simulink model "Model"  (R2020b)
settings: Solver=FixedStepAuto  StartTime=0.0  StopTime=40  FixedStep=0.01  RelTol=1e-3
undefined symbols (not defined in the file or in its folder): DiscIntNeverNeededParam, drv, g, gbox, lqr_integral, lqr_nominal, ms22g, nlmodel, Nu, Nx, sens, stvar_est, Ts, wheel, x01
settings Model: Creator=Utente  LastModifiedBy=pellizzar1

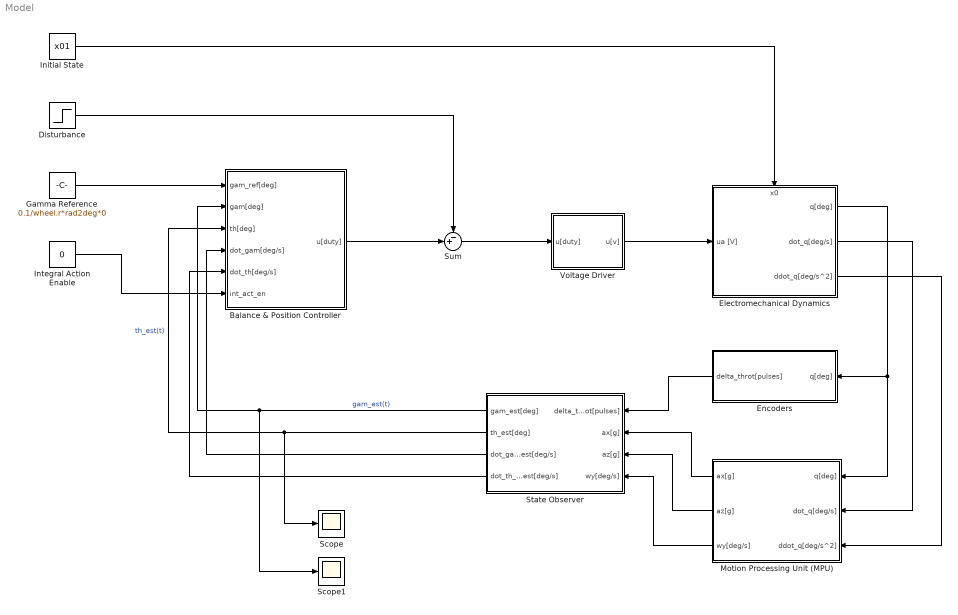
== system Model ==
  Balance & Position Controller : Subsystem
  Disturbance : Step  Time=10  After=5.0/drv.duty2V*0  SampleTime=0
  Electromechanical Dynamics : Subsystem
      settings: PortSchema="{\"entries\":[{\"content\":{\"sides\":[{\"content\":{\"connectorIds\":[\"In1\"]},\"type\":\"ConnectorPlacement.EquallySpacedRectSide\",\"uuid\":\"048a8cca-500e-4f29-b02e-3058ec048dc6\"},{\"content\":{\"connectorIds\":[\"Out1\",\"Out2\",\"Out3\"],\"side\":\"RIGHT\"},\"type\":\"ConnectorPlacement.EquallySpacedRectSide\",\"uuid\":\"804c427c-9fad-47de-8a12-f7821be643d3\"},{\"content\":{\"connectorIds\":[\"In2\"],\"side\":\"TOP\"},\"type\":\"ConnectorPlacement.EquallySpacedRectSide\",\"uuid\":\"0670649b-5041-4c19-9bef-d5e2c260ec4c\"},{\"content\":{\"connectorIds\":[],\"side\":\"HIDDEN\"},\"type\":\"ConnectorPlacement.EquallySpacedRectSide\",\"uuid\":\"076fab11-60d6-4203-9b70-8d32553eb0e9\"}]},\"type\":\"ConnectorPlacement.EquallySpacedConnector\",\"uuid\":\"bba1f46b-97be-4b52-a7cf-094c8f71319b\"}],\"packageUris\":[\"http://schema.mathworks.com/mf0/Connector/R2020b\"],\"version\":\"1.0\"}"
  Encoders : Subsystem
  Gamma Reference : Constant  Value=0.1/wheel.r*rad2deg*0
  Initial State : Constant  Value=x01
  Integral Action Enable : Constant  Value=0
  Motion Processing Unit (MPU) : Subsystem
  Scope : Scope
  Scope1 : Scope
  State Observer : Subsystem
  Sum : Sum  Inputs=-+|
  Voltage Driver : Subsystem
  wires:
  Voltage Driver/1(u[v]) -> Electromechanical Dynamics/1(ua [V])
  Electromechanical Dynamics/2(dot_q[deg/s]) -> Motion Processing Unit (MPU)/2(dot_q[deg/s])
  Electromechanical Dynamics/3(ddot_q[deg/s^2]) -> Motion Processing Unit (MPU)/3(ddot_q[deg/s^2])
  Encoders/1(delta_throt[pulses]) -> State Observer/1(delta_throt[pulses])
  Motion Processing Unit (MPU)/3(wy[deg/s]) -> State Observer/4(wy[deg/s])
  Motion Processing Unit (MPU)/2(az[g]) -> State Observer/3(az[g])
  Motion Processing Unit (MPU)/1(ax[g]) -> State Observer/2(ax[g])
  Balance & Position Controller/1(u[duty]) -> Sum/2
  Disturbance/1 -> Sum/1
  State Observer/4(dot_th_est[deg/s]) -> Balance & Position Controller/5(dot_th[deg/s])
  State Observer/3(dot_gam_est[deg/s]) -> Balance & Position Controller/4(dot_gam[deg/s])
  State Observer/2(th_est[deg]) -> Scope/1, Balance & Position Controller/3(th[deg])  "th_est(t)"
  State Observer/1(gam_est[deg]) -> Scope1/1, Balance & Position Controller/2(gam[deg])  "gam_est(t)"
  Gamma Reference/1 -> Balance & Position Controller/1(gam_ref[deg])
  Electromechanical Dynamics/1(q[deg]) -> Motion Processing Unit (MPU)/1(q[deg]), Encoders/1(q[deg])
  Sum/1 -> Voltage Driver/1(u[duty])
  Initial State/1 -> Electromechanical Dynamics/2(x0)
  Integral Action Enable/1 -> Balance & Position Controller/6(int_act_en)

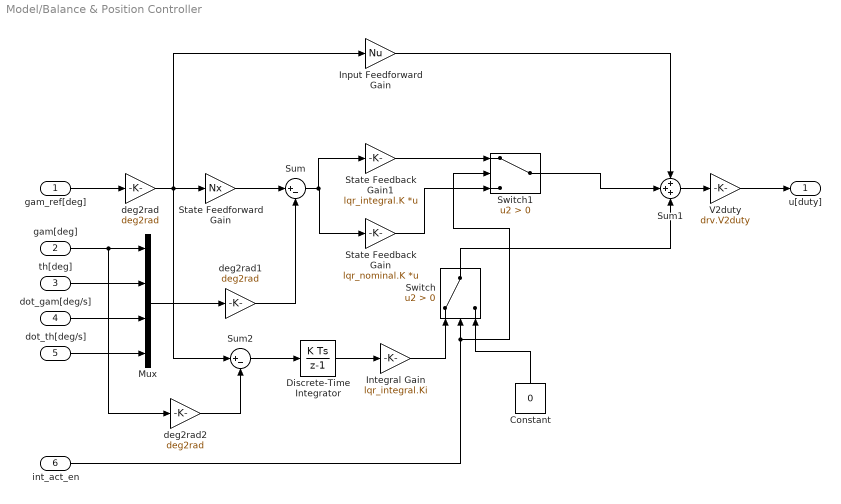
== system Model/Balance & Position Controller ==
  gam_ref[deg] : Inport
  gam[deg] : Inport  Port=2
  th[deg] : Inport  Port=3
  dot_gam[deg/s] : Inport  Port=4
  dot_th[deg/s] : Inport  Port=5
  int_act_en : Inport  Port=6
  Constant : Constant  Value=0
  Discrete-Time Integrator : DiscreteIntegrator  SampleTime=Ts  ICPrevOutput=DiscIntNeverNeededParam  ICPrevScaledInput=DiscIntNeverNeededParam
  Input Feedforward Gain : Gain  Gain=Nu
  Integral Gain : Gain  Gain=lqr_integral.Ki
  Mux : Mux
  State Feedback Gain : Gain  Gain=lqr_nominal.K  Multiplication=Matrix(K*u)
  State Feedback Gain1 : Gain  Gain=lqr_integral.K  Multiplication=Matrix(K*u)
  State Feedforward Gain : Gain  Gain=Nx
  Sum : Sum  Inputs=|+-
  Sum1 : Sum  Inputs=+++
  Sum2 : Sum  Inputs=|+-
  Switch : Switch  Criteria=u2 > Threshold
  Switch1 : Switch  Criteria=u2 > Threshold
  V2duty : Gain  Gain=drv.V2duty
  deg2rad : Gain  Gain=deg2rad
  deg2rad1 : Gain  Gain=deg2rad
  deg2rad2 : Gain  Gain=deg2rad
  u[duty] : Outport
  wires:
  Mux/1 -> deg2rad1/1
  Sum1/1 -> V2duty/1
  th[deg]/1 -> Mux/2
  deg2rad/1 -> Sum2/1, Input Feedforward Gain/1, State Feedforward Gain/1
  dot_gam[deg/s]/1 -> Mux/3
  Input Feedforward Gain/1 -> Sum1/1
  V2duty/1 -> u[duty]/1
  gam_ref[deg]/1 -> deg2rad/1
  gam[deg]/1 -> deg2rad2/1, Mux/1
  dot_th[deg/s]/1 -> Mux/4
  State Feedforward Gain/1 -> Sum/1
  deg2rad1/1 -> Sum/2
  Sum/1 -> State Feedback Gain1/1, State Feedback Gain/1
  Sum2/1 -> Discrete-Time Integrator/1
  deg2rad2/1 -> Sum2/2
  Discrete-Time Integrator/1 -> Integral Gain/1
  Integral Gain/1 -> Switch/1
  Constant/1 -> Switch/3
  int_act_en/1 -> Switch1/2, Switch/2
  State Feedback Gain/1 -> Switch1/3
  Switch1/1 -> Sum1/2
  State Feedback Gain1/1 -> Switch1/1
  Switch/1 -> Sum1/3

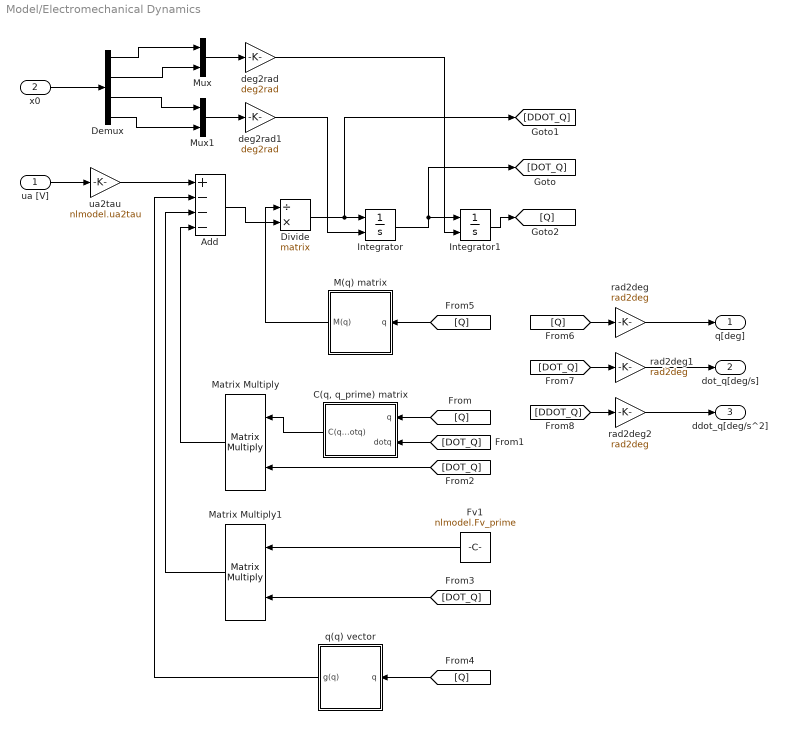
== system Model/Electromechanical Dynamics ==
  ua [V] : Inport
  x0 : Inport  Port=2
  Add : Sum  Inputs=+---
  "C(q, q_prime) matrix" : Subsystem
  Demux : Demux
  Divide : Product  Inputs=/*  Multiplication=Matrix(*)
  Fv1 : Constant  Value=nlmodel.Fv_prime  VectorParams1D=off
  Integrator : Integrator  InitialConditionSource=external
  Integrator1 : Integrator  InitialConditionSource=external  InitialCondition=[0;pi/36]
  M(q) matrix : Subsystem
  Matrix Multiply : Product  Multiplication=Matrix(*)
  Matrix Multiply1 : Product  Multiplication=Matrix(*)
  Mux : Mux  Inputs=2
  Mux1 : Mux  Inputs=2
  deg2rad : Gain  Gain=deg2rad
  deg2rad1 : Gain  Gain=deg2rad
  q(q) vector : Subsystem
  rad2deg : Gain  Gain=rad2deg
  rad2deg1 : Gain  Gain=rad2deg
  rad2deg2 : Gain  Gain=rad2deg
  ua2tau : Gain  Gain=nlmodel.ua2tau
  q[deg] : Outport
  dot_q[deg/s] : Outport  Port=2
  ddot_q[deg/s^2] : Outport  Port=3
  wires:
  Integrator/1 -> [DOT_Q], Integrator1/1
  [Q] -> M(q) matrix/1(q)
  [Q] -> rad2deg/1
  Matrix Multiply1/1 -> Add/3
  rad2deg2/1 -> ddot_q[deg/s^2]/1
  Fv1/1 -> Matrix Multiply1/1
  rad2deg/1 -> q[deg]/1
  Integrator1/1 -> [Q]
  rad2deg1/1 -> dot_q[deg/s]/1
  Matrix Multiply/1 -> Add/4
  Divide/1 -> [DDOT_Q], Integrator/1
  q(q) vector/1(g(q)) -> Add/2
  ua [V]/1 -> ua2tau/1
  ua2tau/1 -> Add/1
  [DOT_Q] -> rad2deg1/1
  [DOT_Q] -> Matrix Multiply/2
  [Q] -> q(q) vector/1(q)
  [DDOT_Q] -> rad2deg2/1
  [DOT_Q] -> "C(q, q_prime) matrix"/2(dotq)
  [Q] -> "C(q, q_prime) matrix"/1(q)
  "C(q, q_prime) matrix"/1("C(q, dotq)") -> Matrix Multiply/1
  M(q) matrix/1(M(q)) -> Divide/1
  Add/1 -> Divide/2
  [DOT_Q] -> Matrix Multiply1/2
  Demux/1 -> Mux/1
  Demux/4 -> Mux1/2
  x0/1 -> Demux/1
  Demux/2 -> Mux/2
  Demux/3 -> Mux1/1
  Mux1/1 -> deg2rad1/1
  Mux/1 -> deg2rad/1
  deg2rad/1 -> Integrator1/2
  deg2rad1/1 -> Integrator/2

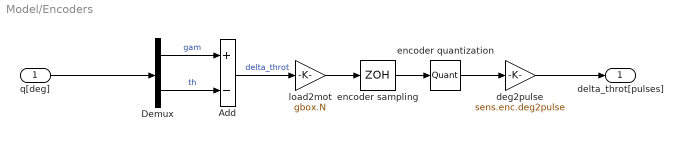
== system Model/Encoders ==
  q[deg] : Inport
  Add : Sum  Inputs=+-
  Demux : Demux  Outputs=2
  deg2pulse : Gain  Gain=sens.enc.deg2pulse
  encoder quantization : Quantizer  QuantizationInterval=sens.enc.pulse2deg
  encoder sampling : ZeroOrderHold  SampleTime=Ts
  load2mot : Gain  Gain=gbox.N
  delta_throt[pulses] : Outport
  wires:
  Add/1 -> load2mot/1  "delta_throt"
  encoder sampling/1 -> encoder quantization/1
  load2mot/1 -> encoder sampling/1
  encoder quantization/1 -> deg2pulse/1
  Demux/2 -> Add/2  "th"
  deg2pulse/1 -> delta_throt[pulses]/1
  q[deg]/1 -> Demux/1
  Demux/1 -> Add/1  "gam"

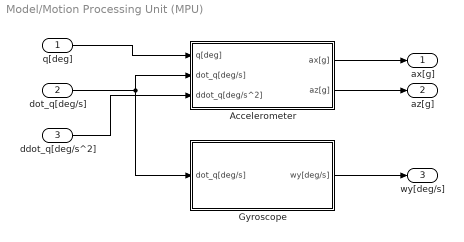
== system Model/Motion Processing Unit (MPU) ==
  q[deg] : Inport
  dot_q[deg/s] : Inport  Port=2
  ddot_q[deg/s^2] : Inport  Port=3
  Accelerometer : Subsystem
  Gyroscope : Subsystem
  ax[g] : Outport
  az[g] : Outport  Port=2
  wy[deg/s] : Outport  Port=3
  wires:
  ddot_q[deg/s^2]/1 -> Accelerometer/3(ddot_q[deg/s^2])
  Accelerometer/1(ax[g]) -> ax[g]/1
  q[deg]/1 -> Accelerometer/1("q[deg] ")
  dot_q[deg/s]/1 -> Gyroscope/1("dot_q[deg/s] "), Accelerometer/2(dot_q[deg/s])
  Gyroscope/1(wy[deg/s]) -> wy[deg/s]/1
  Accelerometer/2(az[g]) -> az[g]/1

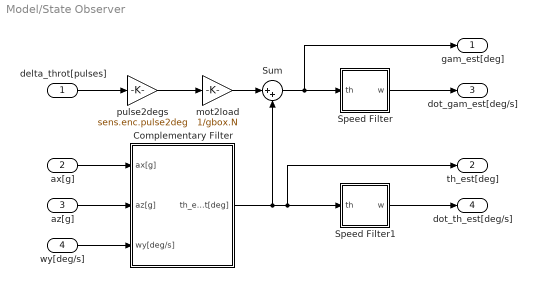
== system Model/State Observer ==
  delta_throt[pulses] : Inport
  ax[g] : Inport  Port=2
  az[g] : Inport  Port=3
  wy[deg/s] : Inport  Port=4
  Complementary Filter : Subsystem
  Speed Filter : Subsystem
  Speed Filter1 : Subsystem
  Sum : Sum  Inputs=|++
  mot2load : Gain  Gain=1/gbox.N
  pulse2degs : Gain  Gain=sens.enc.pulse2deg
  gam_est[deg] : Outport
  th_est[deg] : Outport  Port=2
  dot_gam_est[deg/s] : Outport  Port=3
  dot_th_est[deg/s] : Outport  Port=4
  wires:
  Complementary Filter/1(th_est[deg]) -> th_est[deg]/1, Speed Filter1/1(th), Sum/2
  delta_throt[pulses]/1 -> pulse2degs/1
  ax[g]/1 -> Complementary Filter/1(ax[g])
  az[g]/1 -> Complementary Filter/2(az[g])
  mot2load/1 -> Sum/1
  wy[deg/s]/1 -> Complementary Filter/3(wy[deg/s])
  Speed Filter/1(w) -> dot_gam_est[deg/s]/1
  Speed Filter1/1(w) -> dot_th_est[deg/s]/1
  pulse2degs/1 -> mot2load/1
  Sum/1 -> gam_est[deg]/1, Speed Filter/1(th)

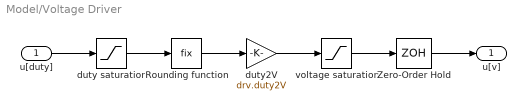
== system Model/Voltage Driver ==
  u[duty] : Inport
  Rounding function : Rounding  Operator=fix
  Zero-Order Hold : ZeroOrderHold  SampleTime=Ts
  duty saturation : Saturate  UpperLimit=drv.dutymax  LowerLimit=-drv.dutymax
  duty2V : Gain  Gain=drv.duty2V
  voltage saturation : Saturate  UpperLimit=drv.Vbus  LowerLimit=-drv.Vbus
  u[v] : Outport
  wires:
  Zero-Order Hold/1 -> u[v]/1
  u[duty]/1 -> duty saturation/1
  duty saturation/1 -> Rounding function/1
  voltage saturation/1 -> Zero-Order Hold/1
  duty2V/1 -> voltage saturation/1
  Rounding function/1 -> duty2V/1

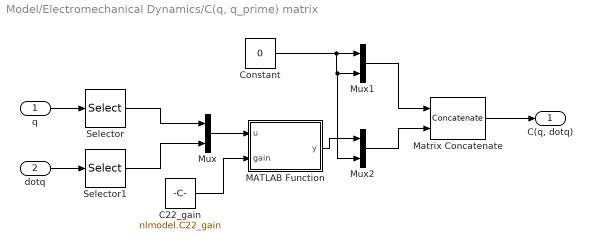
== system Model/Electromechanical Dynamics/C(q, q_prime) matrix ==
  q : Inport
  dotq : Inport  Port=2
  C22_gain : Constant  Value=nlmodel.C22_gain
  Constant : Constant  Value=0
  MATLAB Function : MATLAB Function  TreatAsAtomicUnit=on
  Matrix Concatenate : Concatenate  Mode=Multidimensional array  ConcatenateDimension=2
  Mux : Mux  Inputs=2
  Mux1 : Mux  Inputs=2
  Mux2 : Mux  Inputs=2
  Selector : Selector  InputPortWidth=2  IndexOptions=Index vector (dialog)  Indices=2  OutputSizes=1
  Selector1 : Selector  InputPortWidth=2  IndexOptions=Index vector (dialog)  Indices=2  OutputSizes=1
  "C(q, dotq)" : Outport
  wires:
  Constant/1 -> Mux2/2, Mux1/2, Mux1/1
  Mux2/1 -> Matrix Concatenate/2
  dotq/1 -> Selector1/1
  q/1 -> Selector/1
  Matrix Concatenate/1 -> "C(q, dotq)"/1
  Mux1/1 -> Matrix Concatenate/1
  Selector/1 -> Mux/1
  Selector1/1 -> Mux/2
  Mux/1 -> MATLAB Function/1(u)
  MATLAB Function/1(y) -> Mux2/1
  C22_gain/1 -> MATLAB Function/2(gain)

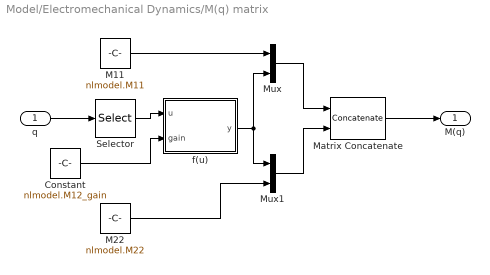
== system Model/Electromechanical Dynamics/M(q) matrix ==
  q : Inport
  Constant : Constant  Value=nlmodel.M12_gain
  M11 : Constant  Value=nlmodel.M11
  M22 : Constant  Value=nlmodel.M22
  Matrix Concatenate : Concatenate  Mode=Multidimensional array  ConcatenateDimension=2
  Mux : Mux  Inputs=2
  Mux1 : Mux  Inputs=2
  Selector : Selector  InputPortWidth=2  IndexOptions=Index vector (dialog)  Indices=2  OutputSizes=1
  f(u) : MATLAB Function  TreatAsAtomicUnit=on
  M(q) : Outport
  wires:
  Mux/1 -> Matrix Concatenate/1
  Selector/1 -> f(u)/1(u)
  M22/1 -> Mux1/2
  f(u)/1(y) -> Mux/2, Mux1/1
  q/1 -> Selector/1
  Matrix Concatenate/1 -> M(q)/1
  Mux1/1 -> Matrix Concatenate/2
  M11/1 -> Mux/1
  Constant/1 -> f(u)/2(gain)

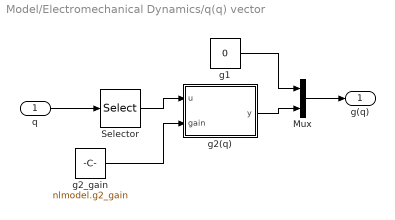
== system Model/Electromechanical Dynamics/q(q) vector ==
  q : Inport
  Mux : Mux  Inputs=2
  Selector : Selector  InputPortWidth=2  IndexOptions=Index vector (dialog)  Indices=2  OutputSizes=1
  g1 : Constant  Value=0
  g2(q) : MATLAB Function  TreatAsAtomicUnit=on
  g2_gain : Constant  Value=nlmodel.g2_gain
  g(q) : Outport
  wires:
  g1/1 -> Mux/1
  Mux/1 -> g(q)/1
  g2(q)/1(y) -> Mux/2
  q/1 -> Selector/1
  Selector/1 -> g2(q)/1(u)
  g2_gain/1 -> g2(q)/2(gain)

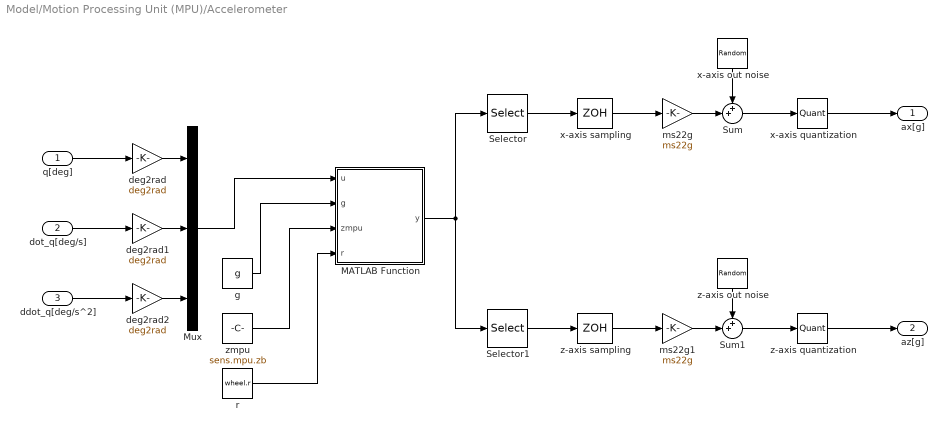
== system Model/Motion Processing Unit (MPU)/Accelerometer ==
  "q[deg] " : Inport
  dot_q[deg/s] : Inport  Port=2
  ddot_q[deg/s^2] : Inport  Port=3
  MATLAB Function : MATLAB Function  TreatAsAtomicUnit=on
  Mux : Mux  Inputs=3
  Selector : Selector  InputPortWidth=2  IndexOptions=Index vector (dialog)  Indices=1  OutputSizes=1
  Selector1 : Selector  InputPortWidth=2  IndexOptions=Index vector (dialog)  Indices=2  OutputSizes=1
  Sum : Sum  Inputs=++|
  Sum1 : Sum  Inputs=++|
  deg2rad : Gain  Gain=deg2rad
  deg2rad1 : Gain  Gain=deg2rad
  deg2rad2 : Gain  Gain=deg2rad
  g : Constant  Value=g
  ms22g : Gain  Gain=ms22g
  ms22g1 : Gain  Gain=ms22g
  r : Constant  Value=wheel.r
  x-axis out noise : RandomNumber  Variance=sens.mpu.acc.noisevar  SampleTime=0.1
  x-axis quantization : Quantizer  QuantizationInterval=sens.mpu.acc.LSB2g
  x-axis sampling : ZeroOrderHold  SampleTime=-1
  z-axis out noise : RandomNumber  Variance=sens.mpu.acc.noisevar  SampleTime=0.1
  z-axis quantization : Quantizer  QuantizationInterval=sens.mpu.acc.LSB2g
  z-axis sampling : ZeroOrderHold  SampleTime=-1
  zmpu : Constant  Value=sens.mpu.zb
  ax[g] : Outport
  az[g] : Outport  Port=2
  wires:
  x-axis sampling/1 -> ms22g/1
  z-axis quantization/1 -> az[g]/1
  deg2rad1/1 -> Mux/2
  x-axis quantization/1 -> ax[g]/1
  ms22g/1 -> Sum/2
  dot_q[deg/s]/1 -> deg2rad1/1
  ms22g1/1 -> Sum1/2
  Sum/1 -> x-axis quantization/1
  Sum1/1 -> z-axis quantization/1
  z-axis out noise/1 -> Sum1/1
  z-axis sampling/1 -> ms22g1/1
  x-axis out noise/1 -> Sum/1
  Mux/1 -> MATLAB Function/1(u)
  Selector1/1 -> z-axis sampling/1
  deg2rad2/1 -> Mux/3
  ddot_q[deg/s^2]/1 -> deg2rad2/1
  deg2rad/1 -> Mux/1
  "q[deg] "/1 -> deg2rad/1
  g/1 -> MATLAB Function/2(g)
  zmpu/1 -> MATLAB Function/3(zmpu)
  r/1 -> MATLAB Function/4(r)
  Selector/1 -> x-axis sampling/1
  MATLAB Function/1(y) -> Selector1/1, Selector/1

== system Model/Motion Processing Unit (MPU)/Gyroscope ==
  "dot_q[deg/s] " : Inport
  Sum2 : Sum  Inputs=++|
  selector : Selector  InputPortWidth=2  IndexOptions=Index vector (dialog)  Indices=[2]  OutputSizes=1
  y-axis out noise : RandomNumber  Variance=sens.mpu.gyro.noisevar  SampleTime=0.1
  y-axis quantization : Quantizer  QuantizationInterval=sens.mpu.gyro.LSB2degs
  y-axis sampling : ZeroOrderHold  SampleTime=-1
  wy[deg/s] : Outport
  wires:
  Sum2/1 -> y-axis quantization/1
  y-axis out noise/1 -> Sum2/1
  y-axis quantization/1 -> wy[deg/s]/1
  selector/1 -> y-axis sampling/1
  y-axis sampling/1 -> Sum2/2
  "dot_q[deg/s] "/1 -> selector/1

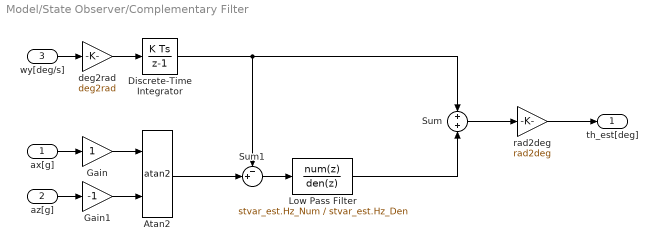
== system Model/State Observer/Complementary Filter ==
  ax[g] : Inport
  az[g] : Inport  Port=2
  wy[deg/s] : Inport  Port=3
  Atan2 : Trigonometry  Operator=atan2
  Discrete-Time Integrator : DiscreteIntegrator  SampleTime=Ts  ICPrevOutput=DiscIntNeverNeededParam  ICPrevScaledInput=DiscIntNeverNeededParam
  Gain : Gain
  Gain1 : Gain  Gain=-1
  "Low Pass Filter " : DiscreteTransferFcn  Numerator=stvar_est.Hz_Num  Denominator=stvar_est.Hz_Den
  Sum : Sum  Inputs=+|+
  Sum1 : Sum  Inputs=-+|
  deg2rad : Gain  Gain=deg2rad
  rad2deg : Gain  Gain=rad2deg
  th_est[deg] : Outport
  wires:
  ax[g]/1 -> Gain/1
  deg2rad/1 -> Discrete-Time Integrator/1
  wy[deg/s]/1 -> deg2rad/1
  Atan2/1 -> Sum1/2
  Gain1/1 -> Atan2/2
  Gain/1 -> Atan2/1
  az[g]/1 -> Gain1/1
  rad2deg/1 -> th_est[deg]/1
  Sum/1 -> rad2deg/1
  Discrete-Time Integrator/1 -> Sum1/1, Sum/1
  Sum1/1 -> "Low Pass Filter "/1
  "Low Pass Filter "/1 -> Sum/2

== system Model/State Observer/Speed Filter ==
  th : Inport
  Real Derivator : DiscreteTransferFcn  Numerator=[1 0 0 -1]  Denominator=[3*Ts 0 0 0]  SampleTime=Ts
  w : Outport
  wires:
  Real Derivator/1 -> w/1
  th/1 -> Real Derivator/1

== system Model/State Observer/Speed Filter1 ==
  th : Inport
  Real Derivator : DiscreteTransferFcn  Numerator=[1 0 0 -1]  Denominator=[3*Ts 0 0 0]  SampleTime=Ts
  w : Outport
  wires:
  Real Derivator/1 -> w/1
  th/1 -> Real Derivator/1

== matlab function Model/Electromechanical Dynamics/C(q, q_prime) matrix/MATLAB Function ==
  data: u input; y output; gain input
function y = C22(u, gain)
theta = u(1);
theta_dot = u(2);
y = gain*sin(theta)*theta_dot;

== matlab function Model/Electromechanical Dynamics/M(q) matrix/f(u) ==
  data: u input; y output; gain input
function y = f(u, gain)
y = gain*cos(u);

== matlab function Model/Electromechanical Dynamics/q(q) vector/g2(q) ==
  data: u input; y output; gain input
function y = f(u, gain)

y = gain*sin(u);

== matlab function Model/Motion Processing Unit (MPU)/Accelerometer/MATLAB Function ==
  data: u input; y output; g input; zmpu input; r input
function y = fcn(u, g, zmpu, r)
theta = u(2);
dot_theta = u(4);
ddot_theta = u(6);
ddot_gamma = u(5);
y = [r*ddot_gamma*cos(theta)+zmpu*ddot_theta+g*sin(theta);r*ddot_gamma*sin(theta)-zmpu*dot_theta*dot_theta-g*cos(theta)];
